simulink model "JFFLZhPID"  (Simulink 8.3)
settings: Solver=ode4  StartTime=0.0  StopTime=1200.0  FixedStep=20  RelTol=1e-3
undefined symbols (not defined in the file or in its folder): DiscIntNeverNeededParam
settings Model: Creator=Zhu Supeng  LastModifiedBy=Zhu Supeng
settings DataIOCC: SignalLoggingName=sigsOut
settings DebuggingCC: SaveWithParameterizedLinksMsg=none  SignalResolutionControl=TryResolveAllWithWarning  SolverPrmCheckMsg=none  MultiTaskDSMMsg=warning  MultiTaskCondExecSysMsg=none  StateNameClashWarn=none
settings HardwareCC: TargetUnknown=on
settings RTWCC: IncludeERTFirstTime=on

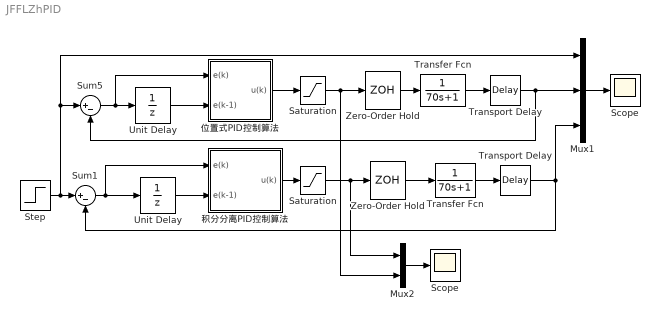
== system JFFLZhPID ==
  Mux1 : Mux  Inputs=3
  Mux2 : Mux  Inputs=2
  Saturation : Saturate  UpperLimit=10  LowerLimit=-10
  "Saturation " : Saturate  UpperLimit=10  LowerLimit=-10
  "Scope " : Scope
      settings: YMin=0  YMax=1  SaveName=JFFLZhPID  MaxDataPoints=500000
  "Scope  " : Scope
      settings: YMin=0  YMax=1  SaveName=JFFLZhPIDu  MaxDataPoints=500000
  Step : Step  Time=0  SampleTime=20
  Sum1 : Sum  Inputs=|+-  SaturateOnIntegerOverflow=on
  Sum5 : Sum  Inputs=|+-  SaturateOnIntegerOverflow=on
  Transfer Fcn : TransferFcn  Denominator=[70 1]
  "Transfer Fcn " : TransferFcn  Denominator=[70 1]
  Transport Delay : TransportDelay  DelayTime=80
  "Transport Delay " : TransportDelay  DelayTime=80
  Unit Delay : UnitDelay  SampleTime=20
  "Unit Delay " : UnitDelay  SampleTime=20
  Zero-Order Hold : ZeroOrderHold  SampleTime=20
  "Zero-Order Hold " : ZeroOrderHold  SampleTime=20
  "位置式PID控制算法 " : Subsystem
  积分分离PID控制算法 : Subsystem
  wires:
  "位置式PID控制算法 "/1(u(k)) -> Saturation/1
  Transfer Fcn/1 -> Transport Delay/1
  Zero-Order Hold/1 -> Transfer Fcn/1
  Transport Delay/1 -> Sum5/2, Mux1/2
  Unit Delay/1 -> "位置式PID控制算法 "/2(e(k-1))
  Sum5/1 -> Unit Delay/1, "位置式PID控制算法 "/1(e(k))
  Step/1 -> Sum1/1, Sum5/1, Mux1/1
  积分分离PID控制算法/1(u(k)) -> "Saturation "/1
  "Transport Delay "/1 -> Mux1/3, Sum1/2
  "Unit Delay "/1 -> 积分分离PID控制算法/2(e(k-1))
  Sum1/1 -> 积分分离PID控制算法/1(e(k)), "Unit Delay "/1
  Mux1/1 -> "Scope "/1
  "Transfer Fcn "/1 -> "Transport Delay "/1
  "Zero-Order Hold "/1 -> "Transfer Fcn "/1
  Saturation/1 -> Zero-Order Hold/1, Mux2/2
  "Saturation "/1 -> "Zero-Order Hold "/1, Mux2/1
  Mux2/1 -> "Scope  "/1

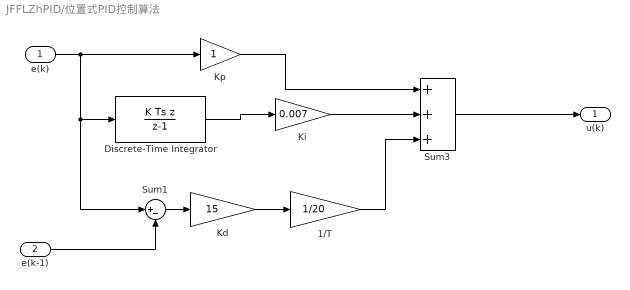
== system JFFLZhPID/位置式PID控制算法  ==
  e(k) : Inport
  e(k-1) : Inport  Port=2
  1/T : Gain  Gain=1/20  SaturateOnIntegerOverflow=on  OutDataTypeStr=Inherit: Same as input  ParamDataTypeStr=Inherit: Same as input
  Discrete-Time Integrator : DiscreteIntegrator  IntegratorMethod=Integration: Backward Euler  SampleTime=20  ICPrevOutput=DiscIntNeverNeededParam  ICPrevScaledInput=DiscIntNeverNeededParam
  Kd : Gain  Gain=15  SaturateOnIntegerOverflow=on  OutDataTypeStr=Inherit: Same as input  ParamDataTypeStr=Inherit: Same as input
  Ki : Gain  Gain=0.007  SaturateOnIntegerOverflow=on  OutDataTypeStr=Inherit: Same as input  ParamDataTypeStr=Inherit: Same as input
  Kp : Gain  SaturateOnIntegerOverflow=on  OutDataTypeStr=Inherit: Same as input  ParamDataTypeStr=Inherit: Same as input
  Sum1 : Sum  Inputs=|+-  SaturateOnIntegerOverflow=on
  Sum3 : Sum  Inputs=+++  SaturateOnIntegerOverflow=on
  u(k) : Outport
  wires:
  Sum1/1 -> Kd/1
  e(k)/1 -> Kp/1, Sum1/1, Discrete-Time Integrator/1
  Kp/1 -> Sum3/1
  Ki/1 -> Sum3/2
  Sum3/1 -> u(k)/1
  Kd/1 -> 1/T/1
  1/T/1 -> Sum3/3
  e(k-1)/1 -> Sum1/2
  Discrete-Time Integrator/1 -> Ki/1

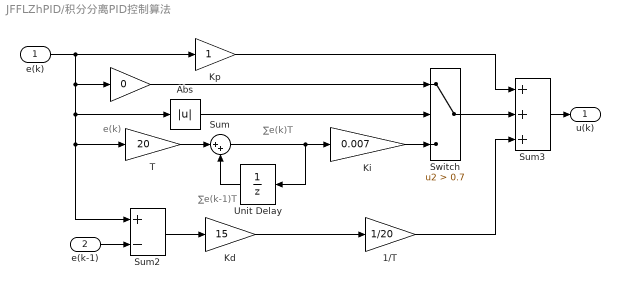
== system JFFLZhPID/积分分离PID控制算法 ==
  note: e(k)
  note: ∑e(k)T
  note: ∑e(k-1)T
  e(k) : Inport
  e(k-1) : Inport  Port=2
  "    " : Gain  Gain=0  SaturateOnIntegerOverflow=on  OutDataTypeStr=Inherit: Same as input  ParamDataTypeStr=Inherit: Same as input
  1/T : Gain  Gain=1/20  SaturateOnIntegerOverflow=on  OutDataTypeStr=Inherit: Same as input  ParamDataTypeStr=Inherit: Same as input
  Abs : Abs  SaturateOnIntegerOverflow=on
  Kd : Gain  Gain=15  SaturateOnIntegerOverflow=on  OutDataTypeStr=Inherit: Same as input  ParamDataTypeStr=Inherit: Same as input
  Ki : Gain  Gain=0.007  SaturateOnIntegerOverflow=on  OutDataTypeStr=Inherit: Same as input  ParamDataTypeStr=Inherit: Same as input
  Kp : Gain  SaturateOnIntegerOverflow=on  OutDataTypeStr=Inherit: Same as input  ParamDataTypeStr=Inherit: Same as input
  Sum : Sum  Inputs=|++  SaturateOnIntegerOverflow=on
  Sum2 : Sum  Inputs=+-  SaturateOnIntegerOverflow=on
  Sum3 : Sum  Inputs=+++  SaturateOnIntegerOverflow=on
  Switch : Switch  Criteria=u2 > Threshold  Threshold=0.7  SaturateOnIntegerOverflow=on  InputSameDT=on
  T : Gain  Gain=20  SaturateOnIntegerOverflow=on  OutDataTypeStr=Inherit: Same as input  ParamDataTypeStr=Inherit: Same as input
  Unit Delay : UnitDelay  SampleTime=20
  u(k) : Outport
  wires:
  Ki/1 -> Switch/3
  Abs/1 -> Switch/2
  "    "/1 -> Switch/1
  Switch/1 -> Sum3/2
  e(k-1)/1 -> Sum2/2
  Sum3/1 -> u(k)/1
  Kp/1 -> Sum3/1
  e(k)/1 -> Abs/1, Sum2/1, T/1, "    "/1, Kp/1
  Sum2/1 -> Kd/1
  Kd/1 -> 1/T/1
  1/T/1 -> Sum3/3
  Sum/1 -> Unit Delay/1, Ki/1
  Unit Delay/1 -> Sum/2
  T/1 -> Sum/1
